simulink model "DOUBLESUPLMMODEL"  (R2022b)
settings: Solver=VariableStepAuto  StartTime=0.0  StopTime=10.0  RelTol=1e-3
libraries: fl_lib x23, nesl_utility x5
settings Model: Creator=andre.pianca  LastModifiedBy=andre.pianca

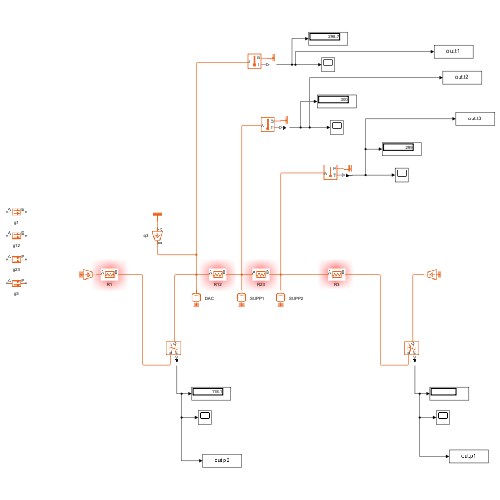
[thumbnail: Simulink's stored preview of the top-level diagram]
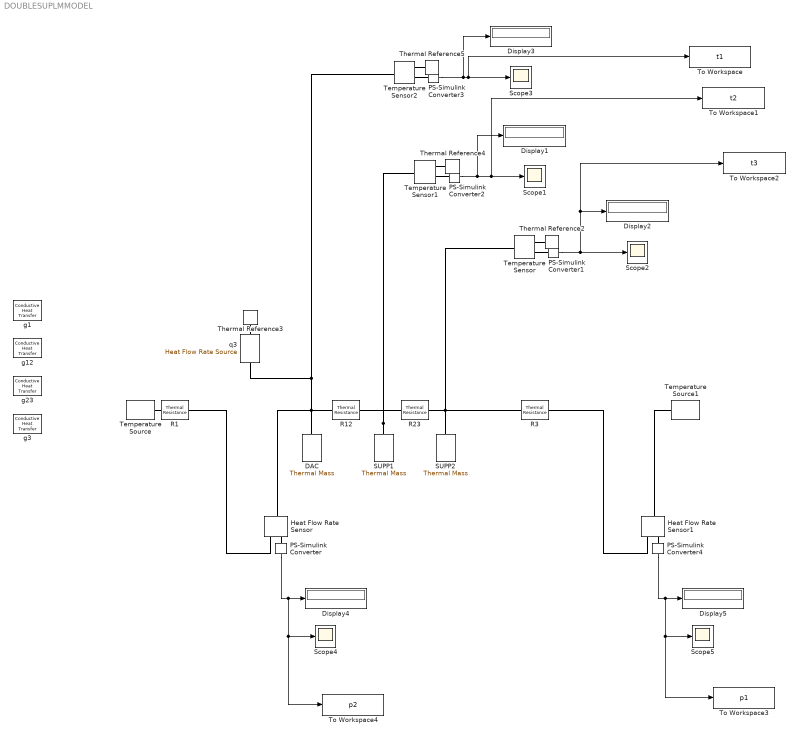
== system DOUBLESUPLMMODEL ==
  DAC : fl_lib/Thermal/Thermal Elements/Thermal Mass  mass=0.432 kg  sp_heat=295.3784090389102 J/(K*kg)  num_ports=foundation.enum.numPorts2.one  T_specify=off  T_priority=High  T=300 K  T_nominal_specify=off  T_nominal_unit=K  T_nominal_value=1  Q_specify=off  Q_priority=None  Q=0 W  Q_nominal_specify=off  Q_nominal_unit=W  Q_nominal_value=1
  Display{1..5} (5 alike) : Display
  Heat Flow Rate Sensor : fl_lib/Thermal/Thermal Sensors/Heat Flow Rate Sensor
  Heat Flow Rate Sensor1 : fl_lib/Thermal/Thermal Sensors/Heat Flow Rate Sensor
  PS-Simulink Converter{,1..4} (5 alike) : nesl_utility/PS-Simulink Converter  PhysicalDomain=network_engine_domain  SubClassName=ps_output  LeftPortType=input  RightPortType=output  PseudoPeriodic=off  Frequencies=[]  VectorFormat=inherit  Unit=inherit  AffineConversion=off
  R1 : fl_lib/Thermal/Thermal Elements/Thermal Resistance  resistance=R1 K/W  T_specify=off  T_priority=None  T=0 K  T_nominal_specify=off  T_nominal_unit=K  T_nominal_value=1  Q_specify=off  Q_priority=None  Q=0 W  Q_nominal_specify=off  Q_nominal_unit=W  Q_nominal_value=1
  R12 : fl_lib/Thermal/Thermal Elements/Thermal Resistance  resistance=R12 K/W  T_specify=off  T_priority=None  T=0 K  T_nominal_specify=off  T_nominal_unit=K  T_nominal_value=1  Q_specify=off  Q_priority=None  Q=0 W  Q_nominal_specify=off  Q_nominal_unit=W  Q_nominal_value=1
  R23 : fl_lib/Thermal/Thermal Elements/Thermal Resistance  resistance=R23 K/W  T_specify=off  T_priority=None  T=0 K  T_nominal_specify=off  T_nominal_unit=K  T_nominal_value=1  Q_specify=off  Q_priority=None  Q=0 W  Q_nominal_specify=off  Q_nominal_unit=W  Q_nominal_value=1
  R3 : fl_lib/Thermal/Thermal Elements/Thermal Resistance  resistance=R3 K/W  T_specify=off  T_priority=None  T=0 K  T_nominal_specify=off  T_nominal_unit=K  T_nominal_value=1  Q_specify=off  Q_priority=None  Q=0 W  Q_nominal_specify=off  Q_nominal_unit=W  Q_nominal_value=1
  SUPP1 : fl_lib/Thermal/Thermal Elements/Thermal Mass  mass=0.332 kg  sp_heat=351.62703271694176 J/(K*kg)  num_ports=foundation.enum.numPorts2.one  T_specify=off  T_priority=High  T=300 K  T_nominal_specify=off  T_nominal_unit=K  T_nominal_value=1  Q_specify=off  Q_priority=None  Q=0 W  Q_nominal_specify=off  Q_nominal_unit=W  Q_nominal_value=1
  SUPP2 : fl_lib/Thermal/Thermal Elements/Thermal Mass  mass=0.332 kg  sp_heat=351.62703271694176 J/(K*kg)  num_ports=foundation.enum.numPorts2.one  T_specify=off  T_priority=High  T=300 K  T_nominal_specify=off  T_nominal_unit=K  T_nominal_value=1  Q_specify=off  Q_priority=None  Q=0 W  Q_nominal_specify=off  Q_nominal_unit=W  Q_nominal_value=1
  Scope{1..5} (5 alike) : Scope
  Temperature Sensor : fl_lib/Thermal/Thermal Sensors/Temperature Sensor
  Temperature Sensor1 : fl_lib/Thermal/Thermal Sensors/Temperature Sensor
  Temperature Sensor2 : fl_lib/Thermal/Thermal Sensors/Temperature Sensor
  Temperature Source : fl_lib/Thermal/Thermal Sources/Temperature Source  temperature=4.2 K
  Temperature Source1 : fl_lib/Thermal/Thermal Sources/Temperature Source  temperature=40 K
  Thermal Reference{2..5} (4 alike) : fl_lib/Thermal/Thermal Elements/Thermal Reference
  To Workspace : ToWorkspace  VariableName=t1  SaveFormat=Timeseries  SampleTime=-1
  To Workspace1 : ToWorkspace  VariableName=t2  SaveFormat=Timeseries  SampleTime=-1
  To Workspace2 : ToWorkspace  VariableName=t3  SaveFormat=Timeseries  SampleTime=-1
  To Workspace3 : ToWorkspace  VariableName=p1  SaveFormat=Timeseries  SampleTime=-1
  To Workspace4 : ToWorkspace  VariableName=p2  SaveFormat=Timeseries  SampleTime=-1
  g{1,3,12,23} (4 alike) : fl_lib/Thermal/Thermal Elements/Conductive Heat Transfer  thermal_type=foundation.enum.ConstantVariableTabulated.Constant  wall_geometry=foundation.enum.ConductionWallGeometry.Planar  area=1e-4 m^2  thickness=0.1 m  d_in=0.05 m  d_out=0.1 m  L=1 m  th_cond_min=10 W/(K*m)  th_cond=401 W/(K*m)  th_cond_TLU=[413, 401, 392, 383, 371, 357, 342] W/(K*m)  temp_TLU=[200, 273, 400, 600, 800, 1000, 1200] K  T_specify=off  T_priority=None  T=0 K  T_nominal_specify=off  T_nominal_unit=K  T_nominal_value=1  Q_specify=off  Q_priority=None  Q=0 W  Q_nominal_specify=off  Q_nominal_unit=W  Q_nominal_value=1
  q3 : fl_lib/Thermal/Thermal Sources/Heat Flow Rate Source  heat_flow=10e-3 W
      settings: InternalSimscapePortConfiguration="{\"Bottom\":[],\"Left\":[{\"id\":\"B\",\"label\":\"B\",\"type\":\"foundation.thermal.thermal\"}],\"Right\":[{\"id\":\"A\",\"label\":\"A\",\"type\":\"foundation.thermal.thermal\"}],\"Top\":[]}"
  wires:
  PS-Simulink Converter2/1 -> Display1/1, To Workspace1/1, Scope1/1
  PS-Simulink Converter1/1 -> To Workspace2/1, Display2/1, Scope2/1
  PS-Simulink Converter3/1 -> Display3/1, To Workspace/1, Scope3/1
  PS-Simulink Converter/1 -> To Workspace4/1, Scope4/1, Display4/1
  PS-Simulink Converter4/1 -> To Workspace3/1, Scope5/1, Display5/1
  connections:
  R1/LConn1 -- Temperature Source/LConn1
  SUPP1/LConn1 -- R23/LConn1 -- R12/RConn1 -- Temperature Sensor1/LConn1
  R1/RConn1 -- Heat Flow Rate Sensor/RConn2
  Thermal Reference3/LConn1 -- q3/RConn1
  q3/LConn1 -- Temperature Sensor2/LConn1 -- R12/LConn1 -- Heat Flow Rate Sensor/LConn1 -- DAC/LConn1
  PS-Simulink Converter/LConn1 -- Heat Flow Rate Sensor/RConn1
  PS-Simulink Converter1/LConn1 -- Temperature Sensor/RConn2
  Thermal Reference2/LConn1 -- Temperature Sensor/RConn1
  SUPP2/LConn1 -- R3/LConn1 -- R23/RConn1 -- Temperature Sensor/LConn1
  Thermal Reference4/LConn1 -- Temperature Sensor1/RConn1
  PS-Simulink Converter2/LConn1 -- Temperature Sensor1/RConn2
  Thermal Reference5/LConn1 -- Temperature Sensor2/RConn1
  PS-Simulink Converter3/LConn1 -- Temperature Sensor2/RConn2
  R3/RConn1 -- Heat Flow Rate Sensor1/RConn2
  PS-Simulink Converter4/LConn1 -- Heat Flow Rate Sensor1/RConn1
  Heat Flow Rate Sensor1/LConn1 -- Temperature Source1/LConn1
